simulink model "DC_Motor_Model"  (R2020b)
settings: Solver=VariableStepAuto  StartTime=0.0  StopTime=10.0  RelTol=1e-3
values from neighbouring files (symbols this model uses):
  B = input('Enter the value of Damping coefficient B=')    [Ajith007MechanicalSys.m]    (also in EX10 (1).m = intput('Enter Damping Constant: '); EX10.m = 0.1; MechSys1st.m = input('Enter the value for Damping coefficient B='); MechSys2nd.m = input('Enter the value for Damper B='))
  J = 0.01    [EX10.m]    (also in Untitled.m)
  Kb = 0.01    [EX10.m]
  Kt = 0.01    [EX10.m]
  La = 0.5    [EX10.m]
  Ra = 1    [EX10.m]
settings Model: Creator=Madhumitha Joe  LastModifiedBy=ajith

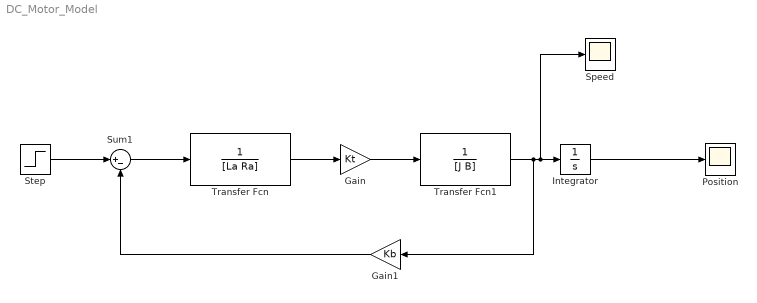
== system DC_Motor_Model ==
  Gain : Gain  Gain=Kt
  Gain1 : Gain  Gain=Kb
  Integrator : Integrator
  Position : Scope
  Speed : Scope
  Step : Step  SampleTime=0
  Sum1 : Sum  Inputs=|+-
  Transfer Fcn : TransferFcn  Denominator=[La Ra]
  Transfer Fcn1 : TransferFcn  Denominator=[J B]
  wires:
  Integrator/1 -> Position/1
  Gain1/1 -> Sum1/2
  Sum1/1 -> Transfer Fcn/1
  Transfer Fcn1/1 -> Gain1/1, Speed/1, Integrator/1
  Gain/1 -> Transfer Fcn1/1
  Transfer Fcn/1 -> Gain/1
  Step/1 -> Sum1/1
